simulink model "comparing_controllers"  (R2020a)
settings: Solver=VariableStepAuto  StartTime=0.0  StopTime=50  RelTol=1e-3
libraries: aerolibutil x20, sharedutil x10, slctrlblks x6
(part 1 of 3)
settings Model: Creator=Sebas  LastModifiedBy=Sebas
settings SolverCC: ZeroCrossAlgorithm=Adaptive
settings DebuggingCC: MaskedZcDiagnostic=none  IgnoredZcDiagnostic=none

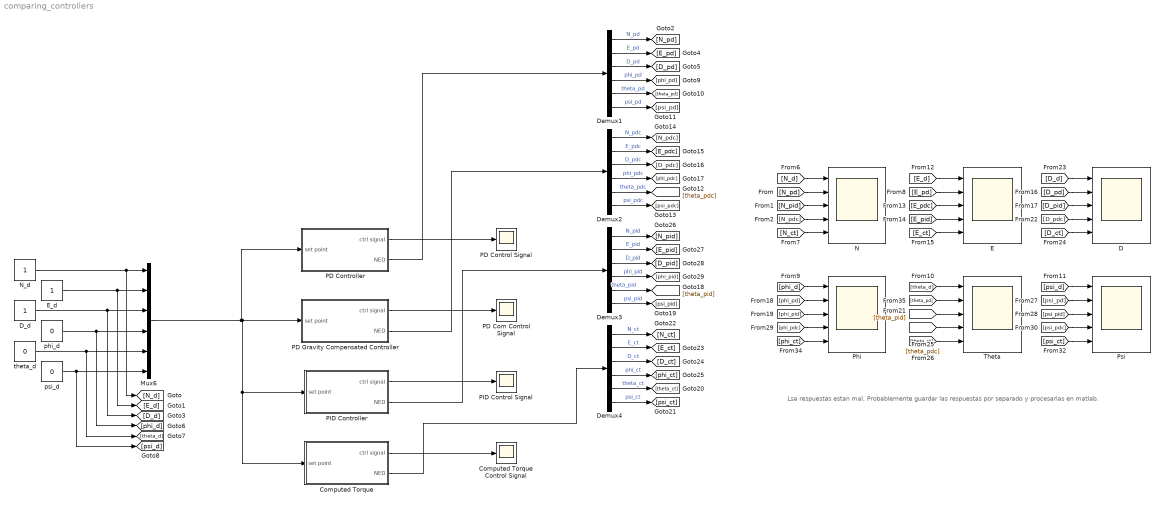
== system comparing_controllers ==
  note: Lsa respuestas estan mal. Probablemente guardar las respuestas por separado y procesarlas en matlab.
  Computed Torque : Subsystem
  Computed Torque Control Signal : Scope
  D : Scope  NumInputPorts=5
  D_d : Constant
  Demux{1..4} (4 alike) : Demux  Outputs=6
  E : Scope  NumInputPorts=5
  E_d : Constant
  Mux6 : Mux  Inputs=6
  N : Scope  NumInputPorts=5
  N_d : Constant
  PD Com Control Signal : Scope
  PD Control Signal : Scope
  PD Controller : Subsystem
  PD Gravity Compensated Controller : Subsystem
  PID Control Signal : Scope
  PID Controller : Subsystem
  Phi : Scope  NumInputPorts=5
  Psi : Scope  NumInputPorts=5
  Theta : Scope  NumInputPorts=5
  phi_d : Constant  Value=0
  psi_d : Constant  Value=0
  theta_d : Constant  Value=0
  wires:
  Demux1/3 -> [D_pd]  "D_pd"
  N_d/1 -> [N_d], Mux6/1
  Demux1/5 -> [theta_pd]  "theta_pd"
  Demux1/1 -> [N_pd]  "N_pd"
  [N_d] -> N/1
  [N_pd] -> N/2
  [N_pid] -> N/3
  D_d/1 -> Mux6/3, [D_d]
  E_d/1 -> [E_d], Mux6/2
  [N_pdc] -> N/4
  Demux1/4 -> [phi_pd]  "phi_pd"
  phi_d/1 -> Mux6/4, [phi_d]
  theta_d/1 -> [theta_d], Mux6/5
  psi_d/1 -> [psi_d], Mux6/6
  Demux1/6 -> [psi_pd]  "psi_pd"
  Demux1/2 -> [E_pd]  "E_pd"
  Mux6/1 -> PD Controller/1(set point), Computed Torque/1(set point), PID Controller/1(set point), PD Gravity Compensated Controller/1(set point)
  PD Controller/1(ctrl signal) -> PD Control Signal/1
  PD Controller/2(NED) -> Demux1/1
  PD Gravity Compensated Controller/1(ctrl signal) -> PD Com Control Signal/1
  PID Controller/1(ctrl signal) -> PID Control Signal/1
  Computed Torque/1(ctrl signal) -> Computed Torque Control Signal/1
  Demux2/6 -> [psi_pdc]  "psi_pdc"
  Demux2/4 -> [phi_pdc]  "phi_pdc"
  Demux2/2 -> [E_pdc]  "E_pdc"
  Demux2/1 -> [N_pdc]  "N_pdc"
  Demux2/5 -> [theta_pdc]  "theta_pdc"
  Demux2/3 -> [D_pdc]  "D_pdc"
  PD Gravity Compensated Controller/2(NED) -> Demux2/1
  Demux3/2 -> [E_pid]  "E_pid"
  Demux3/6 -> [psi_pid]  "psi_pid"
  Demux3/4 -> [phi_pid]  "phi_pid"
  Demux3/1 -> [N_pid]  "N_pid"
  Demux3/5 -> [theta_pid]  "theta_pid"
  Demux3/3 -> [D_pid]  "D_pid"
  Demux4/6 -> [psi_ct]  "psi_ct"
  Demux4/4 -> [phi_ct]  "phi_ct"
  Demux4/1 -> [N_ct]  "N_ct"
  Demux4/5 -> [theta_ct]  "theta_ct"
  Demux4/2 -> [E_ct]  "E_ct"
  Demux4/3 -> [D_ct]  "D_ct"
  PID Controller/2(NED) -> Demux3/1
  Computed Torque/2(NED) -> Demux4/1
  [N_ct] -> N/5
  [E_ct] -> E/5
  [E_pid] -> E/4
  [E_pdc] -> E/3
  [E_pd] -> E/2
  [E_d] -> E/1
  [D_ct] -> D/5
  [D_pd] -> D/2
  [D_pid] -> D/3
  [D_d] -> D/1
  [D_pdc] -> D/4
  [theta_pd] -> Theta/2
  [theta_d] -> Theta/1
  [theta_pdc] -> Theta/4
  [theta_pid] -> Theta/3
  [phi_pdc] -> Phi/4
  [phi_ct] -> Phi/5
  [psi_ct] -> Psi/5
  [psi_pd] -> Psi/2
  [theta_ct] -> Theta/5
  [phi_pd] -> Phi/2
  [psi_pdc] -> Psi/4
  [phi_pid] -> Phi/3
  [psi_d] -> Psi/1
  [psi_pid] -> Psi/3
  [phi_d] -> Phi/1

== system comparing_controllers/Computed Torque ==
  set point : Inport
  Computed Torque Controller : Subsystem
  Terminator : Terminator
  UUV 6DOF Model : Subsystem
  ctrl signal : Outport
  NED : Outport  Port=2
  wires:
  Computed Torque Controller/1(tau) -> ctrl signal/1, UUV 6DOF Model/1(tau)  "ctrl signal"
  UUV 6DOF Model/3(NED) -> NED/1, Computed Torque Controller/2(NED)
  UUV 6DOF Model/1(vel_dot) -> Terminator/1
  set point/1 -> Computed Torque Controller/1(set point)
  UUV 6DOF Model/2(vel) -> Computed Torque Controller/3(vel)

== system comparing_controllers/PD Controller ==
  set point : Inport
  6 DOF PD Controller : Subsystem
  Terminator : Terminator
  Terminator1 : Terminator
  UUV 6DOF Model : Subsystem
  ctrl signal : Outport
  NED : Outport  Port=2
  wires:
  6 DOF PD Controller/1(tau) -> ctrl signal/1, UUV 6DOF Model/1(tau)  "ctrl signal"
  UUV 6DOF Model/2(vel) -> Terminator1/1
  UUV 6DOF Model/3(NED) -> NED/1, 6 DOF PD Controller/2(current)
  UUV 6DOF Model/1(vel_dot) -> Terminator/1
  set point/1 -> 6 DOF PD Controller/1(set point)

== system comparing_controllers/PD Gravity Compensated Controller ==
  set point : Inport
  6 DOF PD Gravity Comp Controller : Subsystem
  Terminator : Terminator
  Terminator1 : Terminator
  UUV 6DOF Model : Subsystem
  ctrl signal : Outport
  NED : Outport  Port=2
  wires:
  UUV 6DOF Model/2(vel) -> Terminator1/1
  UUV 6DOF Model/1(vel_dot) -> Terminator/1
  6 DOF PD Gravity Comp Controller/1(tau) -> ctrl signal/1, UUV 6DOF Model/1(tau)  "ctrl signal"
  UUV 6DOF Model/3(NED) -> NED/1, 6 DOF PD Gravity Comp Controller/2(current)
  set point/1 -> 6 DOF PD Gravity Comp Controller/1(set point)

== system comparing_controllers/PID Controller ==
  set point : Inport
  6 DOF PID Controller : Subsystem
  Terminator : Terminator
  Terminator1 : Terminator
  UUV 6DOF Model : Subsystem
  ctrl signal : Outport
  NED : Outport  Port=2
  wires:
  UUV 6DOF Model/1(vel_dot) -> Terminator/1
  6 DOF PID Controller/1(tau) -> ctrl signal/1, UUV 6DOF Model/1(tau)  "ctrl signal"
  set point/1 -> 6 DOF PID Controller/1(set point)
  UUV 6DOF Model/3(NED) -> NED/1, 6 DOF PID Controller/2(current)
  UUV 6DOF Model/2(vel) -> Terminator1/1

== system comparing_controllers/Computed Torque/Computed Torque Controller ==
  set point : Inport
  NED : Inport  Port=2
  vel : Inport  Port=3
  6 PD + fb linearization Controllers : Subsystem  mask(6 Degrees-of-freedom P-D Controller){surge_kd=0.35, surge_kp=0.7, sway_kd=0.7, sway_kp=0.6, heave_kd=0.2, heave_kp=0.7, roll_kd=1.3, roll_kp=10, pitch_kd=0.05, pitch_kp=0.2, yaw_kd=1.2, yaw_kp=3}
      mask prompts: surge_kd "Surge K derivative"; surge_kp "Surge K proportional"; sway_kd "Sway K derivative"; sway_kp "Sway K proportional"; heave_kd "Heave K derivative"; heave_kp "Heave K proportional"; roll_kd "Roll K derivative"; roll_kp "Roll K proportional"; pitch_kd "Pitch K derivative"; pitch_kp "Pitch K proportional"; yaw_kd "Yaw K derivative"; yaw_kp "Yaw K proportional"
      mask help: Implementation of 6 PD controllers for each degree of freedom
      mask DialogControl ParameterGroupVar Prompt: Gains
  Constant : Constant  Value=0
  Derivative : Derivative  Commented=on
  Derivative1 : Derivative  Commented=on
  Signal Specification : SignalSpecification  Dimensions=6
  Thrust allocation : Subsystem
  Transform : Subsystem
  tau : Outport
  wires:
  Transform/1(Out1) -> 6 PD + fb linearization Controllers/1(set point)  "ideal"
  NED/1 -> Transform/2(NED)
  Signal Specification/1 -> tau/1  "ideal"
  Transform/2(Out2) -> 6 PD + fb linearization Controllers/2(current)  "ideal"
  Thrust allocation/1(tau) -> Signal Specification/1
  6 PD + fb linearization Controllers/1(i_tau) -> Thrust allocation/1(ideal_tau)  "ideal_tau"
  vel/1 -> 6 PD + fb linearization Controllers/3(vel)  "ideal"
  set point/1 -> Transform/1(set point)  "ideal"
  Constant/1 -> 6 PD + fb linearization Controllers/4(vel_dot_d)
  Derivative/1 -> Derivative1/1

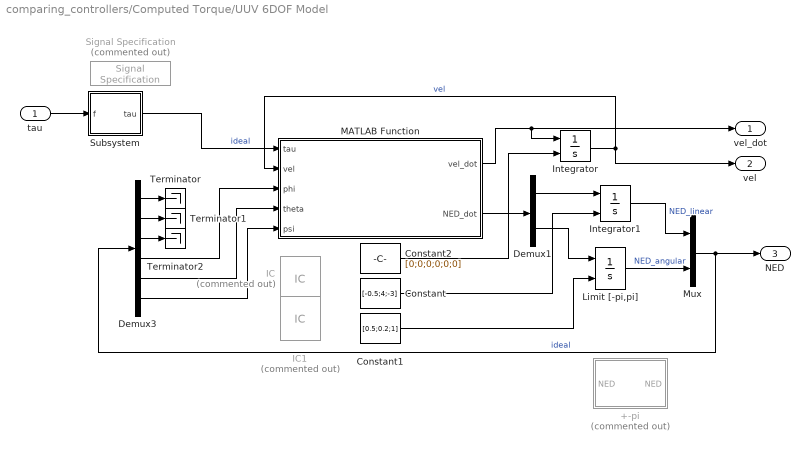
== system comparing_controllers/Computed Torque/UUV 6DOF Model ==
  tau : Inport
  +-pi : MATLAB Function  Commented=on  TreatAsAtomicUnit=on
  Constant : Constant  Value=[-0.5;4;-3]
  Constant1 : Constant  Value=[0.5;0.2;1]
  Constant2 : Constant  Value=[0;0;0;0;0;0]
  Demux1 : Demux  Outputs=2
  Demux3 : Demux  Outputs=6
  IC : InitialCondition  Commented=on  Value=[0;0;0;0;0;0]
  IC1 : InitialCondition  Commented=on  Value=[1;1;1;1;1;1]
  Integrator : Integrator  InitialConditionSource=external
  Integrator1 : Integrator  InitialConditionSource=external
  Limit [-pi,pi] : Integrator  InitialConditionSource=external  WrapState=on
  MATLAB Function : MATLAB Function  TreatAsAtomicUnit=on
  Mux : Mux  Inputs=2
  Signal Specification : SignalSpecification  Commented=on  Dimensions=6
  Subsystem : Subsystem
  Terminator : Terminator
  Terminator1 : Terminator
  Terminator2 : Terminator
  vel_dot : Outport
  vel : Outport  Port=2
  NED : Outport  Port=3
  wires:
  Constant/1 -> Integrator1/2
  Constant1/1 -> Limit [-pi,pi]/2
  Constant2/1 -> Integrator/2
  MATLAB Function/2(NED_dot) -> Demux1/1
  Demux1/1 -> Integrator1/1
  Demux1/2 -> Limit [-pi,pi]/1
  Limit [-pi,pi]/1 -> Mux/2  "NED_angular"
  tau/1 -> Subsystem/1(f)
  Subsystem/1(tau) -> MATLAB Function/1(tau)  "ideal"
  Demux3/3 -> Terminator2/1
  Demux3/1 -> Terminator/1
  Demux3/2 -> Terminator1/1
  Integrator1/1 -> Mux/1  "NED_linear"
  Demux3/6 -> MATLAB Function/5(psi)
  Demux3/5 -> MATLAB Function/4(theta)
  Demux3/4 -> MATLAB Function/3(phi)
  Integrator/1 -> MATLAB Function/2(vel), vel/1  "vel"
  MATLAB Function/1(vel_dot) -> Integrator/1, vel_dot/1
  Mux/1 -> NED/1, Demux3/1  "ideal"

== system comparing_controllers/PD Controller/6 DOF PD Controller ==
  set point : Inport
  current : Inport  Port=2
  6 PD Controllers : Subsystem  mask(6 Degrees-of-freedom P-D Controller){surge_kd=25, surge_kp=15, sway_kd=30, sway_kp=12, heave_kd=7, heave_kp=10, roll_kd=0.6, roll_kp=5, pitch_kd=0, pitch_kp=5, yaw_kd=4.5, yaw_kp=5}
      mask prompts: surge_kd "Surge K derivative"; surge_kp "Surge K proportional"; sway_kd "Sway K derivative"; sway_kp "Sway K proportional"; heave_kd "Heave K derivative"; heave_kp "Heave K proportional"; roll_kd "Roll K derivative"; roll_kp "Roll K proportional"; pitch_kd "Pitch K derivative"; pitch_kp "Pitch K proportional"; yaw_kd "Yaw K derivative"; yaw_kp "Yaw K proportional"
      mask help: Implementation of 6 PD controllers for each degree of freedom
      mask DialogControl ParameterGroupVar Prompt: Gains
  Signal Specification : SignalSpecification  Dimensions=6
  Subsystem : Subsystem  Commented=on
  Thrust allocation : Subsystem
  Transform : Subsystem
  tau : Outport
  wires:
  6 PD Controllers/1(i_tau) -> Thrust allocation/1(ideal_tau)  "ideal_tau"
  Thrust allocation/1(tau) -> Signal Specification/1
  set point/1 -> Transform/1(In1)
  current/1 -> Transform/2(NED)
  Transform/1(Out1) -> 6 PD Controllers/1(set point)
  Transform/2(Out2) -> 6 PD Controllers/2(current)
  Signal Specification/1 -> tau/1  "ideal"

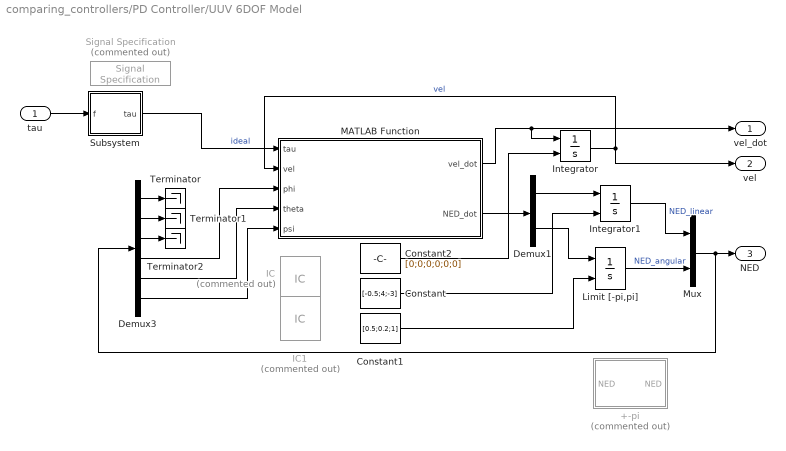
== system comparing_controllers/PD Controller/UUV 6DOF Model ==
  tau : Inport
  +-pi : MATLAB Function  Commented=on  TreatAsAtomicUnit=on
  Constant : Constant  Value=[-0.5;4;-3]
  Constant1 : Constant  Value=[0.5;0.2;1]
  Constant2 : Constant  Value=[0;0;0;0;0;0]
  Demux1 : Demux  Outputs=2
  Demux3 : Demux  Outputs=6
  IC : InitialCondition  Commented=on  Value=[0;0;0;0;0;0]
  IC1 : InitialCondition  Commented=on  Value=[1;1;1;1;1;1]
  Integrator : Integrator  InitialConditionSource=external
  Integrator1 : Integrator  InitialConditionSource=external
  Limit [-pi,pi] : Integrator  InitialConditionSource=external  WrapState=on
  MATLAB Function : MATLAB Function  TreatAsAtomicUnit=on
  Mux : Mux  Inputs=2
  Signal Specification : SignalSpecification  Commented=on  Dimensions=6
  Subsystem : Subsystem
  Terminator : Terminator
  Terminator1 : Terminator
  Terminator2 : Terminator
  vel_dot : Outport
  vel : Outport  Port=2
  NED : Outport  Port=3
  wires:
  Constant/1 -> Integrator1/2
  Constant1/1 -> Limit [-pi,pi]/2
  Constant2/1 -> Integrator/2
  MATLAB Function/2(NED_dot) -> Demux1/1
  Demux1/1 -> Integrator1/1
  Demux1/2 -> Limit [-pi,pi]/1
  Limit [-pi,pi]/1 -> Mux/2  "NED_angular"
  tau/1 -> Subsystem/1(f)
  Subsystem/1(tau) -> MATLAB Function/1(tau)  "ideal"
  Demux3/3 -> Terminator2/1
  Demux3/1 -> Terminator/1
  Demux3/2 -> Terminator1/1
  Integrator1/1 -> Mux/1  "NED_linear"
  Demux3/6 -> MATLAB Function/5(psi)
  Demux3/5 -> MATLAB Function/4(theta)
  Demux3/4 -> MATLAB Function/3(phi)
  Integrator/1 -> MATLAB Function/2(vel), vel/1  "vel"
  Mux/1 -> NED/1, Demux3/1
  MATLAB Function/1(vel_dot) -> Integrator/1, vel_dot/1

== system comparing_controllers/PD Gravity Compensated Controller/6 DOF PD Gravity Comp Controller ==
  set point : Inport
  current : Inport  Port=2
  6 PD Gravity Comp Controllers : Subsystem  mask(6 Degrees-of-freedom P-D and Gravity Compensator Controller){surge_kd=10, surge_kp=5, sway_kd=10, sway_kp=2.5, heave_kd=10, heave_kp=5, roll_kd=30, roll_kp=5, pitch_kd=30, pitch_kp=0.9, yaw_kd=30, yaw_kp=5}
      mask prompts: surge_kd "Surge K derivative"; surge_kp "Surge K proportional"; sway_kd "Sway K derivative"; sway_kp "Sway K proportional"; heave_kd "Heave K derivative"; heave_kp "Heave K proportional"; roll_kd "Roll K derivative"; roll_kp "Roll K proportional"; pitch_kd "Pitch K derivative"; pitch_kp "Pitch K proportional"; yaw_kd "Yaw K derivative"; yaw_kp "Yaw K proportional"
      mask help: Implementation of 6 PD controllers for each degree of freedom plus a Gravity Compensation
      mask DialogControl ParameterGroupVar Prompt: Gains
  Demux6 : Demux  Commented=on  Outputs=3
  Mux2 : Mux  Commented=on  Inputs=3
  Saturation : Saturate  Commented=on  UpperLimit=70  LowerLimit=-70
  Saturation1 : Saturate  Commented=on  UpperLimit=100  LowerLimit=-100
  Saturation2 : Saturate  Commented=on  UpperLimit=100  LowerLimit=-100
  Signal Specification : SignalSpecification  Dimensions=6
  Subsystem : Subsystem  Commented=on
  Subsystem3 : Subsystem  Commented=on
  Thrust allocation : Subsystem
  Transform : Subsystem
  tau : Outport
  wires:
  6 PD Gravity Comp Controllers/1(i_tau) -> Thrust allocation/1(ideal_tau)  "ideal_tau"
  Thrust allocation/1(tau) -> Signal Specification/1  "ideal_t_sat"
  set point/1 -> Transform/1(In1)
  current/1 -> Transform/2(NED)
  Transform/1(Out1) -> 6 PD Gravity Comp Controllers/1(set point)
  Transform/2(Out2) -> 6 PD Gravity Comp Controllers/2(current)
  Saturation1/1 -> Mux2/1
  Saturation/1 -> Mux2/3
  Demux6/2 -> Saturation2/1
  Demux6/1 -> Saturation1/1
  Saturation2/1 -> Mux2/2
  Demux6/3 -> Saturation/1
  Signal Specification/1 -> tau/1  "ideal"

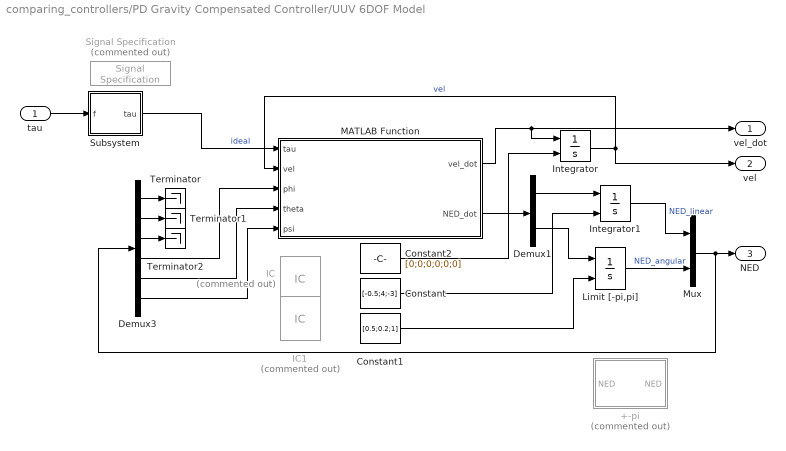
== system comparing_controllers/PD Gravity Compensated Controller/UUV 6DOF Model ==
  tau : Inport
  +-pi : MATLAB Function  Commented=on  TreatAsAtomicUnit=on
  Constant : Constant  Value=[-0.5;4;-3]
  Constant1 : Constant  Value=[0.5;0.2;1]
  Constant2 : Constant  Value=[0;0;0;0;0;0]
  Demux1 : Demux  Outputs=2
  Demux3 : Demux  Outputs=6
  IC : InitialCondition  Commented=on  Value=[0;0;0;0;0;0]
  IC1 : InitialCondition  Commented=on  Value=[1;1;1;1;1;1]
  Integrator : Integrator  InitialConditionSource=external
  Integrator1 : Integrator  InitialConditionSource=external
  Limit [-pi,pi] : Integrator  InitialConditionSource=external  WrapState=on
  MATLAB Function : MATLAB Function  TreatAsAtomicUnit=on
  Mux : Mux  Inputs=2
  Signal Specification : SignalSpecification  Commented=on  Dimensions=6
  Subsystem : Subsystem
  Terminator : Terminator
  Terminator1 : Terminator
  Terminator2 : Terminator
  vel_dot : Outport
  vel : Outport  Port=2
  NED : Outport  Port=3
  wires:
  Constant/1 -> Integrator1/2
  Constant1/1 -> Limit [-pi,pi]/2
  Constant2/1 -> Integrator/2
  MATLAB Function/2(NED_dot) -> Demux1/1
  Demux1/1 -> Integrator1/1
  Demux1/2 -> Limit [-pi,pi]/1
  Limit [-pi,pi]/1 -> Mux/2  "NED_angular"
  tau/1 -> Subsystem/1(f)
  Subsystem/1(tau) -> MATLAB Function/1(tau)  "ideal"
  Demux3/3 -> Terminator2/1
  Demux3/1 -> Terminator/1
  Demux3/2 -> Terminator1/1
  Integrator1/1 -> Mux/1  "NED_linear"
  Demux3/6 -> MATLAB Function/5(psi)
  Demux3/5 -> MATLAB Function/4(theta)
  Demux3/4 -> MATLAB Function/3(phi)
  Integrator/1 -> MATLAB Function/2(vel), vel/1  "vel"
  Mux/1 -> NED/1, Demux3/1
  MATLAB Function/1(vel_dot) -> Integrator/1, vel_dot/1

== system comparing_controllers/PID Controller/6 DOF PID Controller ==
  set point : Inport
  current : Inport  Port=2
  6 PID Controllers : Subsystem  mask(6 Degrees-of-freedom P-I-D Controller){surge_kd=22, surge_kp=13, surge_ki=0, sway_kd=22, sway_kp=7, sway_ki=0, heave_kd=15, heave_kp=7, heave_ki=0.18, roll_kd=0.6, roll_kp=5, roll_ki=0.1, pitch_kd=0, pitch_kp=5, pitch_ki=0.1, yaw_kd=4.5, yaw_kp=5, yaw_ki=0}
      mask prompts: surge_kd "Surge K derivative"; surge_kp "Surge K proportional"; surge_ki "Surge K integral"; sway_kd "Sway K derivative"; sway_kp "Sway K proportional"; sway_ki "Sway K integral"; heave_kd "Heave K derivative"; heave_kp "Heave K proportional"; heave_ki "Heave K integral"; roll_kd "Roll K derivative"; roll_kp "Roll K proportional"; roll_ki "Roll K integral"; pitch_kd "Pitch K derivative"; pitch_kp "Pitch K proportional"; pitch_ki "Pitch K integral"; yaw_kd "Yaw K derivative"; yaw_kp "Yaw K proportional"; yaw_ki "Yaw K integral"
      mask help: Implementation of 6 PID controllers for each degree of freedom
      mask DialogControl ParameterGroupVar Prompt: Gains
  Signal Specification : SignalSpecification  Dimensions=6
  Thrust allocation : Subsystem
  Transform : Subsystem
  tau : Outport
  wires:
  Transform/2(Out2) -> 6 PID Controllers/2(current)
  Thrust allocation/1(tau) -> Signal Specification/1
  Transform/1(Out1) -> 6 PID Controllers/1(set point)
  6 PID Controllers/1(i_tau) -> Thrust allocation/1(ideal_tau)  "ideal_tau"
  Signal Specification/1 -> tau/1  "ideal"
  set point/1 -> Transform/1(set point)
  current/1 -> Transform/2(NED)

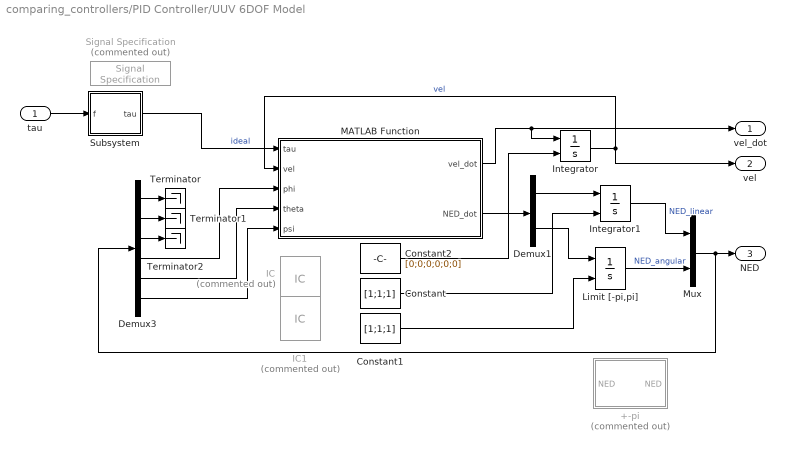
== system comparing_controllers/PID Controller/UUV 6DOF Model ==
  tau : Inport
  +-pi : MATLAB Function  Commented=on  TreatAsAtomicUnit=on
  Constant : Constant  Value=[1;1;1]
  Constant1 : Constant  Value=[1;1;1]
  Constant2 : Constant  Value=[0;0;0;0;0;0]
  Demux1 : Demux  Outputs=2
  Demux3 : Demux  Outputs=6
  IC : InitialCondition  Commented=on  Value=[0;0;0;0;0;0]
  IC1 : InitialCondition  Commented=on  Value=[1;1;1;1;1;1]
  Integrator : Integrator  InitialConditionSource=external
  Integrator1 : Integrator  InitialConditionSource=external
  Limit [-pi,pi] : Integrator  InitialConditionSource=external  WrapState=on
  MATLAB Function : MATLAB Function  TreatAsAtomicUnit=on
  Mux : Mux  Inputs=2
  Signal Specification : SignalSpecification  Commented=on  Dimensions=6
  Subsystem : Subsystem
  Terminator : Terminator
  Terminator1 : Terminator
  Terminator2 : Terminator
  vel_dot : Outport
  vel : Outport  Port=2
  NED : Outport  Port=3
  wires:
  Constant/1 -> Integrator1/2
  Constant1/1 -> Limit [-pi,pi]/2
  Constant2/1 -> Integrator/2
  MATLAB Function/2(NED_dot) -> Demux1/1
  Demux1/1 -> Integrator1/1
  Demux1/2 -> Limit [-pi,pi]/1
  Limit [-pi,pi]/1 -> Mux/2  "NED_angular"
  tau/1 -> Subsystem/1(f)
  Subsystem/1(tau) -> MATLAB Function/1(tau)  "ideal"
  Demux3/3 -> Terminator2/1
  Demux3/1 -> Terminator/1
  Demux3/2 -> Terminator1/1
  Integrator1/1 -> Mux/1  "NED_linear"
  Demux3/6 -> MATLAB Function/5(psi)
  Demux3/5 -> MATLAB Function/4(theta)
  Demux3/4 -> MATLAB Function/3(phi)
  Integrator/1 -> MATLAB Function/2(vel), vel/1  "vel"
  Mux/1 -> NED/1, Demux3/1
  MATLAB Function/1(vel_dot) -> Integrator/1, vel_dot/1

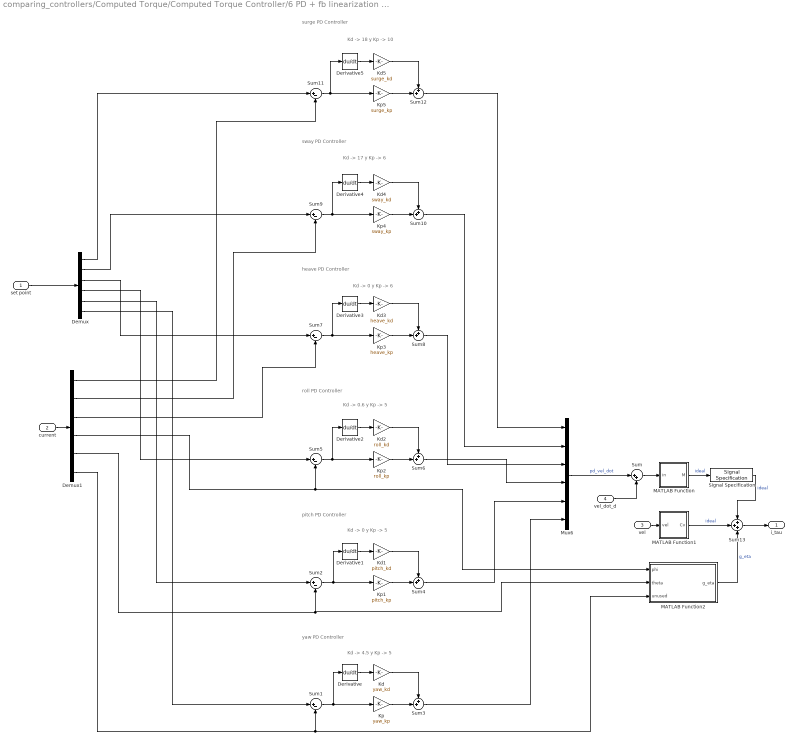
== system comparing_controllers/Computed Torque/Computed Torque Controller/6 PD + fb linearization Controllers ==
  note: surge PD Controller
  note: sway PD Controller
  note: heave PD Controller
  note: roll PD Controller
  note: pitch PD Controller
  note: yaw PD Controller
  note: Kd -> 4.5 y Kp -> 5
  note: Kd -> 0 y Kp -> 5
  note: Kd -> 0.6 y Kp -> 5
  note: Kd -> 0 y Kp -> 6
  note: Kd -> 17 y Kp -> 6
  note: Kd -> 18 y Kp -> 10
  set point : Inport
  current : Inport  Port=2
  vel : Inport  Port=3
  vel_dot_d : Inport  Port=4
  Demux : Demux  Outputs=6
  Demux1 : Demux  Outputs=6
  Derivative{,1..5} (6 alike) : Derivative
  Kd : Gain  Gain=yaw_kd
  Kd1 : Gain  Gain=pitch_kd
  Kd2 : Gain  Gain=roll_kd
  Kd3 : Gain  Gain=heave_kd
  Kd4 : Gain  Gain=sway_kd
  Kd5 : Gain  Gain=surge_kd
  Kp : Gain  Gain=yaw_kp
  Kp1 : Gain  Gain=pitch_kp
  Kp2 : Gain  Gain=roll_kp
  Kp3 : Gain  Gain=heave_kp
  Kp4 : Gain  Gain=sway_kp
  Kp5 : Gain  Gain=surge_kp
  MATLAB Function : MATLAB Function  TreatAsAtomicUnit=on
  MATLAB Function1 : MATLAB Function  TreatAsAtomicUnit=on
  MATLAB Function2 : MATLAB Function  TreatAsAtomicUnit=on
  Mux6 : Mux  Inputs=6
  Signal Specification : SignalSpecification  Dimensions=6
  Sum : Sum  Inputs=|++
  Sum{1..2,5,7,9,11} (6 alike) : Sum  Inputs=|+-
  Sum{3..4,6,8,10,12} (6 alike) : Sum  Inputs=++|
  Sum13 : Sum  Inputs=+++
  i_tau : Outport
  wires:
  Sum8/1 -> Mux6/3
  Sum4/1 -> Mux6/5
  Sum6/1 -> Mux6/4
  Sum3/1 -> Mux6/6
  Sum12/1 -> Mux6/1
  Sum10/1 -> Mux6/2
  Derivative/1 -> Kd/1
  Kp/1 -> Sum3/2
  Kd/1 -> Sum3/1
  Sum1/1 -> Derivative/1, Kp/1
  Sum2/1 -> Kp1/1, Derivative1/1
  Kd1/1 -> Sum4/1
  Kp1/1 -> Sum4/2
  Derivative1/1 -> Kd1/1
  Derivative2/1 -> Kd2/1
  Kp2/1 -> Sum6/2
  Kd2/1 -> Sum6/1
  Sum5/1 -> Derivative2/1, Kp2/1
  Derivative3/1 -> Kd3/1
  Kp3/1 -> Sum8/2
  Kd3/1 -> Sum8/1
  Sum7/1 -> Derivative3/1, Kp3/1
  Derivative4/1 -> Kd4/1
  Kp4/1 -> Sum10/2
  Kd4/1 -> Sum10/1
  Sum9/1 -> Derivative4/1, Kp4/1
  Derivative5/1 -> Kd5/1
  Kp5/1 -> Sum12/2
  Kd5/1 -> Sum12/1
  Sum11/1 -> Derivative5/1, Kp5/1
  current/1 -> Demux1/1
  Demux1/1 -> Sum11/2
  set point/1 -> Demux/1
  Demux/1 -> Sum11/1
  Demux/2 -> Sum9/1
  Demux1/2 -> Sum9/2
  Demux/3 -> Sum7/1
  Demux1/3 -> Sum7/2
  Demux/4 -> Sum5/1
  Demux1/4 -> MATLAB Function2/1(phi), Sum5/2
  Demux/5 -> Sum2/1
  Demux1/5 -> MATLAB Function2/2(theta), Sum2/2
  Demux/6 -> Sum1/1
  Demux1/6 -> MATLAB Function2/3(unused), Sum1/2
  Mux6/1 -> Sum/1  "pd_vel_dot"
  Sum/1 -> MATLAB Function/1(in)
  vel_dot_d/1 -> Sum/2
  Sum13/1 -> i_tau/1
  vel/1 -> MATLAB Function1/1(vel)
  MATLAB Function/1(M) -> Signal Specification/1  "ideal"
  MATLAB Function2/1(g_eta) -> Sum13/3  "g_eta"
  MATLAB Function1/1(Cv) -> Sum13/2  "ideal"
  Signal Specification/1 -> Sum13/1  "ideal"

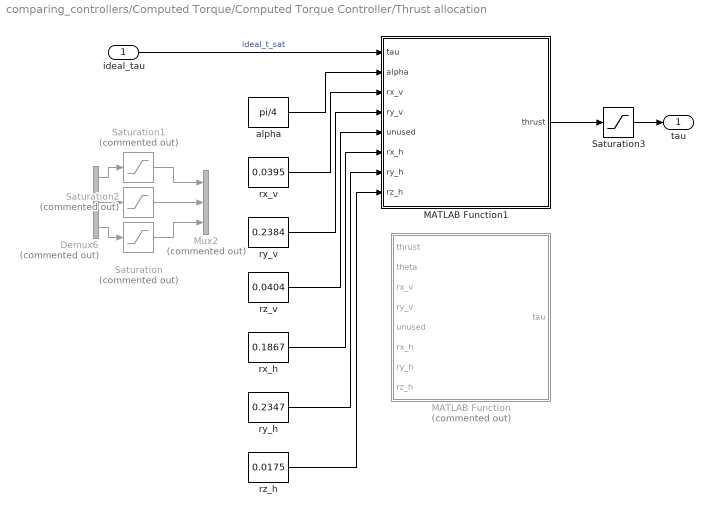
== system comparing_controllers/Computed Torque/Computed Torque Controller/Thrust allocation ==
  ideal_tau : Inport
  Demux6 : Demux  Commented=on  Outputs=3
  MATLAB Function : MATLAB Function  Commented=on  TreatAsAtomicUnit=on
  MATLAB Function1 : MATLAB Function  TreatAsAtomicUnit=on
  Mux2 : Mux  Commented=on  Inputs=3
  Saturation : Saturate  Commented=on  UpperLimit=70  LowerLimit=-70
  Saturation1 : Saturate  Commented=on  UpperLimit=100  LowerLimit=-100
  Saturation2 : Saturate  Commented=on  UpperLimit=100  LowerLimit=-100
  Saturation3 : Saturate  UpperLimit=35  LowerLimit=-35
  alpha : Constant  Value=pi/4
  rx_h : Constant  Value=0.1867
  rx_v : Constant  Value=0.0395
  ry_h : Constant  Value=0.2347
  ry_v : Constant  Value=0.2384
  rz_h : Constant  Value=0.0175
  rz_v : Constant  Value=0.0404
  tau : Outport
  wires:
  ideal_tau/1 -> MATLAB Function1/1(tau)  "ideal_t_sat"
  MATLAB Function1/1(thrust) -> Saturation3/1
  Saturation3/1 -> tau/1
  rx_v/1 -> MATLAB Function1/3(rx_v)
  alpha/1 -> MATLAB Function1/2(alpha)
  rx_h/1 -> MATLAB Function1/6(rx_h)
  ry_h/1 -> MATLAB Function1/7(ry_h)
  rz_h/1 -> MATLAB Function1/8(rz_h)
  ry_v/1 -> MATLAB Function1/4(ry_v)
  rz_v/1 -> MATLAB Function1/5(unused)
  Demux6/2 -> Saturation2/1
  Demux6/3 -> Saturation/1
  Saturation1/1 -> Mux2/1
  Saturation/1 -> Mux2/3
  Demux6/1 -> Saturation1/1
  Saturation2/1 -> Mux2/2

== system comparing_controllers/Computed Torque/Computed Torque Controller/Transform ==
  set point : Inport
  NED : Inport  Port=2
  Demux : Demux  Outputs=2
  Demux1 : Demux  Outputs=2
  Mux1 : Mux  Inputs=2
  Mux2 : Mux  Inputs=2
  Mux3 : Mux  Inputs=2
  Subsystem1 : Subsystem
  Subsystem2 : Subsystem
  Terminator5 : Terminator
  Out1 : Outport
  Out2 : Outport  Port=2
  wires:
  Demux/1 -> Mux2/1
  NED/1 -> Demux1/1, Subsystem1/1(NED)
  set point/1 -> Demux/1
  Demux/2 -> Mux1/2
  Subsystem2/1(pos_body) -> Mux1/1
  Demux1/1 -> Terminator5/1
  Subsystem1/1(pos_body) -> Mux3/1
  Demux1/2 -> Mux2/2, Mux3/2
  Mux2/1 -> Subsystem2/1(NED)
  Mux3/1 -> Out2/1
  Mux1/1 -> Out1/1

== system comparing_controllers/Computed Torque/UUV 6DOF Model/Subsystem ==
  f : Inport
  MATLAB Function1 : MATLAB Function  TreatAsAtomicUnit=on
  rx_h : Constant  Value=0.1867
  rx_v : Constant  Value=0.0395
  ry_h : Constant  Value=0.2347
  ry_v : Constant  Value=0.2384
  rz_h : Constant  Value=0.0175
  rz_v : Constant  Value=0.0404
  theta : Constant  Value=pi/4
  tau : Outport
  wires:
  rz_v/1 -> MATLAB Function1/5(unused)
  ry_h/1 -> MATLAB Function1/7(ry_h)
  f/1 -> MATLAB Function1/1(f)
  MATLAB Function1/1(tau) -> tau/1
  rx_h/1 -> MATLAB Function1/6(rx_h)
  theta/1 -> MATLAB Function1/2(theta)
  rx_v/1 -> MATLAB Function1/3(rx_v)
  rz_h/1 -> MATLAB Function1/8(rz_h)
  ry_v/1 -> MATLAB Function1/4(ry_v)

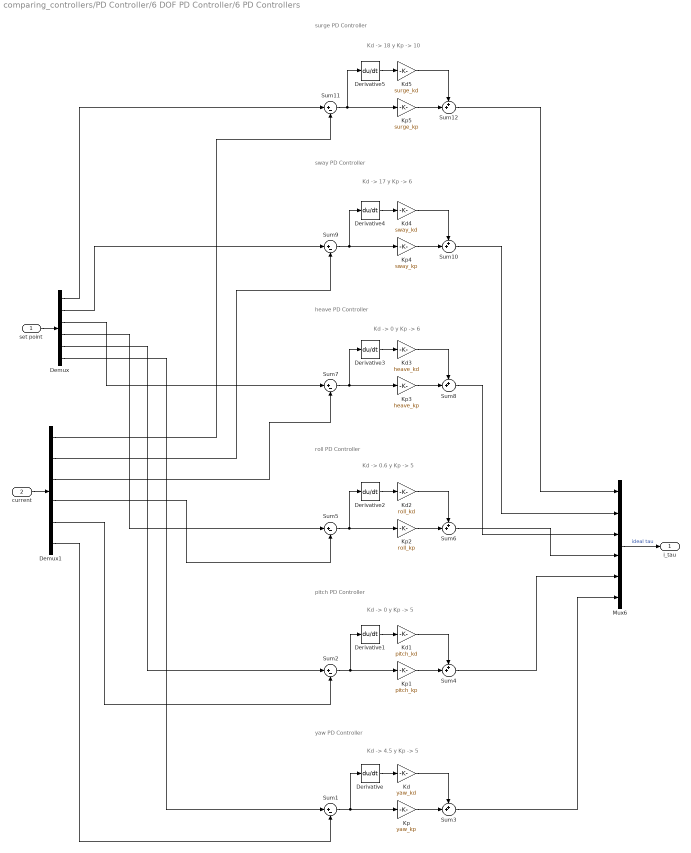
== system comparing_controllers/PD Controller/6 DOF PD Controller/6 PD Controllers ==
  note: surge PD Controller
  note: sway PD Controller
  note: heave PD Controller
  note: roll PD Controller
  note: pitch PD Controller
  note: yaw PD Controller
  note: Kd -> 4.5 y Kp -> 5
  note: Kd -> 0 y Kp -> 5
  note: Kd -> 0.6 y Kp -> 5
  note: Kd -> 0 y Kp -> 6
  note: Kd -> 17 y Kp -> 6
  note: Kd -> 18 y Kp -> 10
  set point : Inport
  current : Inport  Port=2
  Demux : Demux  Outputs=6
  Demux1 : Demux  Outputs=6
  Derivative{,1..5} (6 alike) : Derivative
  Kd : Gain  Gain=yaw_kd
  Kd1 : Gain  Gain=pitch_kd
  Kd2 : Gain  Gain=roll_kd
  Kd3 : Gain  Gain=heave_kd
  Kd4 : Gain  Gain=sway_kd
  Kd5 : Gain  Gain=surge_kd
  Kp : Gain  Gain=yaw_kp
  Kp1 : Gain  Gain=pitch_kp
  Kp2 : Gain  Gain=roll_kp
  Kp3 : Gain  Gain=heave_kp
  Kp4 : Gain  Gain=sway_kp
  Kp5 : Gain  Gain=surge_kp
  Mux6 : Mux  Inputs=6
  Sum{1..2,5,7,9,11} (6 alike) : Sum  Inputs=|+-
  Sum{3..4,6,8,10,12} (6 alike) : Sum  Inputs=++|
  i_tau : Outport
  wires:
  Sum8/1 -> Mux6/3
  Sum4/1 -> Mux6/5
  Sum6/1 -> Mux6/4
  Sum3/1 -> Mux6/6
  Sum12/1 -> Mux6/1
  Sum10/1 -> Mux6/2
  Derivative/1 -> Kd/1
  Kp/1 -> Sum3/2
  Kd/1 -> Sum3/1
  Sum1/1 -> Derivative/1, Kp/1
  Sum2/1 -> Kp1/1, Derivative1/1
  Kd1/1 -> Sum4/1
  Kp1/1 -> Sum4/2
  Derivative1/1 -> Kd1/1
  Derivative2/1 -> Kd2/1
  Kp2/1 -> Sum6/2
  Kd2/1 -> Sum6/1
  Sum5/1 -> Derivative2/1, Kp2/1
  Derivative3/1 -> Kd3/1
  Kp3/1 -> Sum8/2
  Kd3/1 -> Sum8/1
  Sum7/1 -> Derivative3/1, Kp3/1
  Derivative4/1 -> Kd4/1
  Kp4/1 -> Sum10/2
  Kd4/1 -> Sum10/1
  Sum9/1 -> Derivative4/1, Kp4/1
  Derivative5/1 -> Kd5/1
  Kp5/1 -> Sum12/2
  Kd5/1 -> Sum12/1
  Sum11/1 -> Derivative5/1, Kp5/1
  current/1 -> Demux1/1
  Demux1/1 -> Sum11/2
  set point/1 -> Demux/1
  Demux/1 -> Sum11/1
  Demux/2 -> Sum9/1
  Demux1/2 -> Sum9/2
  Demux/3 -> Sum7/1
  Demux1/3 -> Sum7/2
  Demux/4 -> Sum5/1
  Demux1/4 -> Sum5/2
  Demux/5 -> Sum2/1
  Demux1/5 -> Sum2/2
  Demux/6 -> Sum1/1
  Demux1/6 -> Sum1/2
  Mux6/1 -> i_tau/1  "ideal tau"

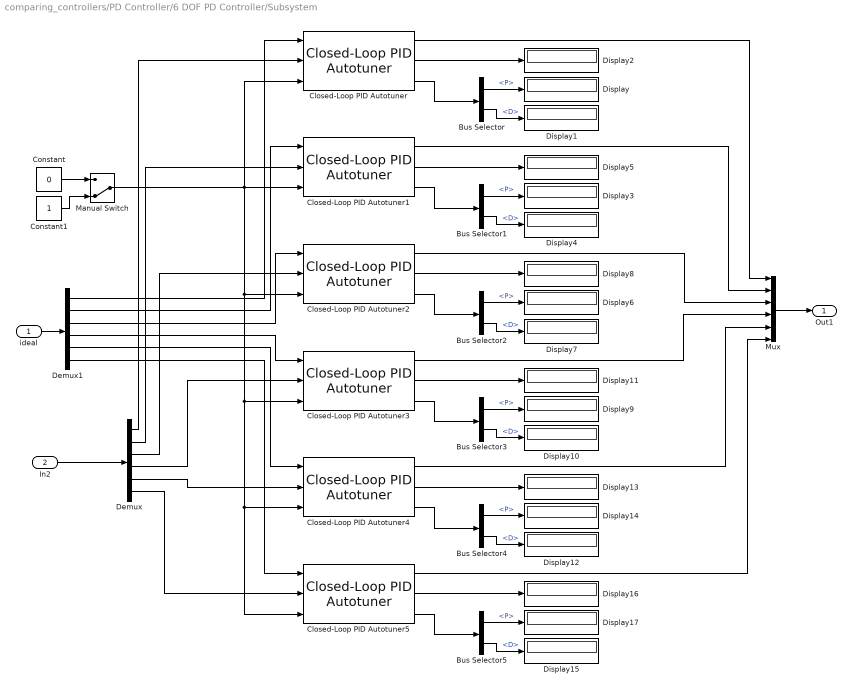
== system comparing_controllers/PD Controller/6 DOF PD Controller/Subsystem ==
  ideal : Inport
  In2 : Inport  Port=2
  Bus Selector{,1..5} (6 alike) : BusSelector  OutputSignals=P,D
  Closed-Loop PID Autotuner{,1..5} (6 alike) : slctrlblks/Closed-Loop PID Autotuner  PIDType=PD  PIDForm=Parallel  TimeDomain=continuous-time  DiscreteTs=0.1  IntegratorFormula=Forward Euler  FilterFormula=Forward Euler  ContinuousTs=0.02  Bandwidth=2/10  UseExternalWC=off  TargetPM=60  UseExternalPM=off  UseExternalAchievedPM=off  PlantType=Integrating  PlantSign=Positive  AmpSine=35  UseExternalAmpSine=off  UseExternalFRD=off  UseExternalU0=off  UseCompanion=off  NotDeployTuningModule=off  UsePLCCoder=off  OutputMode=control action + perturbation  BlockDataType=double  UseConnectedPID=on  blockpath=[]  tunedP=0  tunedI=0  tunedD=0  tunedN=100  tunedPM=0  EstimationWindowSize=3  UseExternalTuningParams=off  OutputChoice=VariantCandD
      settings: SourceProductBaseCode=SD
  Constant : Constant  Value=0
  Constant1 : Constant
  Demux : Demux  Outputs=6
  Demux1 : Demux  Outputs=6
  Display{,1..17} (18 alike) : Display
  Manual Switch : ManualSwitch  CurrentSetting=0
  Mux : Mux  Inputs=6
  Out1 : Outport
  wires:
  Closed-Loop PID Autotuner2/3 -> Bus Selector2/1
  Closed-Loop PID Autotuner/2 -> Display2/1
  Constant/1 -> Manual Switch/1
  Demux/4 -> Closed-Loop PID Autotuner3/2
  Closed-Loop PID Autotuner/3 -> Bus Selector/1
  Manual Switch/1 -> Closed-Loop PID Autotuner/3, Closed-Loop PID Autotuner5/3, Closed-Loop PID Autotuner4/3, Closed-Loop PID Autotuner3/3, Closed-Loop PID Autotuner2/3, Closed-Loop PID Autotuner1/3
  Closed-Loop PID Autotuner2/1 -> Mux/3
  Closed-Loop PID Autotuner4/2 -> Display13/1
  Bus Selector3/1 -> Display9/1  "<P>"
  Bus Selector4/1 -> Display14/1  "<P>"
  Closed-Loop PID Autotuner3/3 -> Bus Selector3/1
  Bus Selector1/2 -> Display4/1  "<D>"
  Constant1/1 -> Manual Switch/2
  Demux1/1 -> Closed-Loop PID Autotuner/1
  Bus Selector/1 -> Display/1  "<P>"
  Closed-Loop PID Autotuner3/2 -> Display11/1
  ideal/1 -> Demux1/1
  Demux1/6 -> Closed-Loop PID Autotuner5/1
  Demux1/5 -> Closed-Loop PID Autotuner4/1
  Bus Selector3/2 -> Display10/1  "<D>"
  Closed-Loop PID Autotuner1/2 -> Display5/1
  Demux1/4 -> Closed-Loop PID Autotuner3/1
  Bus Selector/2 -> Display1/1  "<D>"
  Demux/2 -> Closed-Loop PID Autotuner1/2
  Demux1/3 -> Closed-Loop PID Autotuner2/1
  Closed-Loop PID Autotuner1/1 -> Mux/2
  Closed-Loop PID Autotuner5/2 -> Display16/1
  Bus Selector4/2 -> Display12/1  "<D>"
  Bus Selector1/1 -> Display3/1  "<P>"
  Closed-Loop PID Autotuner1/3 -> Bus Selector1/1
  Demux1/2 -> Closed-Loop PID Autotuner1/1
  Closed-Loop PID Autotuner5/1 -> Mux/6
  Closed-Loop PID Autotuner4/1 -> Mux/5
  Closed-Loop PID Autotuner3/1 -> Mux/4
  In2/1 -> Demux/1
  Closed-Loop PID Autotuner5/3 -> Bus Selector5/1
  Closed-Loop PID Autotuner/1 -> Mux/1
  Bus Selector5/1 -> Display17/1  "<P>"
  Demux/3 -> Closed-Loop PID Autotuner2/2
  Bus Selector5/2 -> Display15/1  "<D>"
  Demux/5 -> Closed-Loop PID Autotuner4/2
  Bus Selector2/2 -> Display7/1  "<D>"
  Demux/1 -> Closed-Loop PID Autotuner/2
  Bus Selector2/1 -> Display6/1  "<P>"
  Closed-Loop PID Autotuner2/2 -> Display8/1
  Closed-Loop PID Autotuner4/3 -> Bus Selector4/1
  Demux/6 -> Closed-Loop PID Autotuner5/2
  Mux/1 -> Out1/1

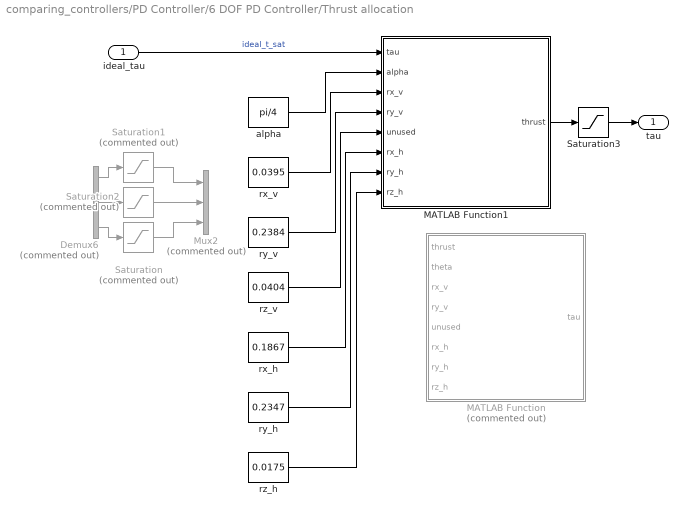
== system comparing_controllers/PD Controller/6 DOF PD Controller/Thrust allocation ==
  ideal_tau : Inport
  Demux6 : Demux  Commented=on  Outputs=3
  MATLAB Function : MATLAB Function  Commented=on  TreatAsAtomicUnit=on
  MATLAB Function1 : MATLAB Function  TreatAsAtomicUnit=on
  Mux2 : Mux  Commented=on  Inputs=3
  Saturation : Saturate  Commented=on  UpperLimit=70  LowerLimit=-70
  Saturation1 : Saturate  Commented=on  UpperLimit=100  LowerLimit=-100
  Saturation2 : Saturate  Commented=on  UpperLimit=100  LowerLimit=-100
  Saturation3 : Saturate  UpperLimit=35  LowerLimit=-35
  alpha : Constant  Value=pi/4
  rx_h : Constant  Value=0.1867
  rx_v : Constant  Value=0.0395
  ry_h : Constant  Value=0.2347
  ry_v : Constant  Value=0.2384
  rz_h : Constant  Value=0.0175
  rz_v : Constant  Value=0.0404
  tau : Outport
  wires:
  ideal_tau/1 -> MATLAB Function1/1(tau)  "ideal_t_sat"
  MATLAB Function1/1(thrust) -> Saturation3/1
  Saturation3/1 -> tau/1
  rx_v/1 -> MATLAB Function1/3(rx_v)
  alpha/1 -> MATLAB Function1/2(alpha)
  rx_h/1 -> MATLAB Function1/6(rx_h)
  ry_h/1 -> MATLAB Function1/7(ry_h)
  rz_h/1 -> MATLAB Function1/8(rz_h)
  ry_v/1 -> MATLAB Function1/4(ry_v)
  rz_v/1 -> MATLAB Function1/5(unused)
  Demux6/2 -> Saturation2/1
  Demux6/3 -> Saturation/1
  Saturation1/1 -> Mux2/1
  Saturation/1 -> Mux2/3
  Demux6/1 -> Saturation1/1
  Saturation2/1 -> Mux2/2

== system comparing_controllers/PD Controller/6 DOF PD Controller/Transform ==
  In1 : Inport
  NED : Inport  Port=2
  Demux : Demux  Outputs=2
  Demux1 : Demux  Outputs=2
  Mux1 : Mux  Inputs=2
  Mux2 : Mux  Inputs=2
  Mux3 : Mux  Inputs=2
  Subsystem1 : Subsystem
  Subsystem2 : Subsystem
  Terminator5 : Terminator
  Out1 : Outport
  Out2 : Outport  Port=2
  wires:
  Demux/1 -> Mux2/1
  NED/1 -> Demux1/1, Subsystem1/1(NED)
  In1/1 -> Demux/1
  Demux/2 -> Mux1/2
  Subsystem2/1(pos_body) -> Mux1/1
  Demux1/1 -> Terminator5/1
  Subsystem1/1(pos_body) -> Mux3/1
  Demux1/2 -> Mux2/2, Mux3/2
  Mux2/1 -> Subsystem2/1(NED)
  Mux3/1 -> Out2/1
  Mux1/1 -> Out1/1

== system comparing_controllers/PD Controller/UUV 6DOF Model/Subsystem ==
  f : Inport
  MATLAB Function1 : MATLAB Function  TreatAsAtomicUnit=on
  rx_h : Constant  Value=0.1867
  rx_v : Constant  Value=0.0395
  ry_h : Constant  Value=0.2347
  ry_v : Constant  Value=0.2384
  rz_h : Constant  Value=0.0175
  rz_v : Constant  Value=0.0404
  theta : Constant  Value=pi/4
  tau : Outport
  wires:
  rz_v/1 -> MATLAB Function1/5(unused)
  ry_h/1 -> MATLAB Function1/7(ry_h)
  f/1 -> MATLAB Function1/1(f)
  MATLAB Function1/1(tau) -> tau/1
  rx_h/1 -> MATLAB Function1/6(rx_h)
  theta/1 -> MATLAB Function1/2(theta)
  rx_v/1 -> MATLAB Function1/3(rx_v)
  rz_h/1 -> MATLAB Function1/8(rz_h)
  ry_v/1 -> MATLAB Function1/4(ry_v)

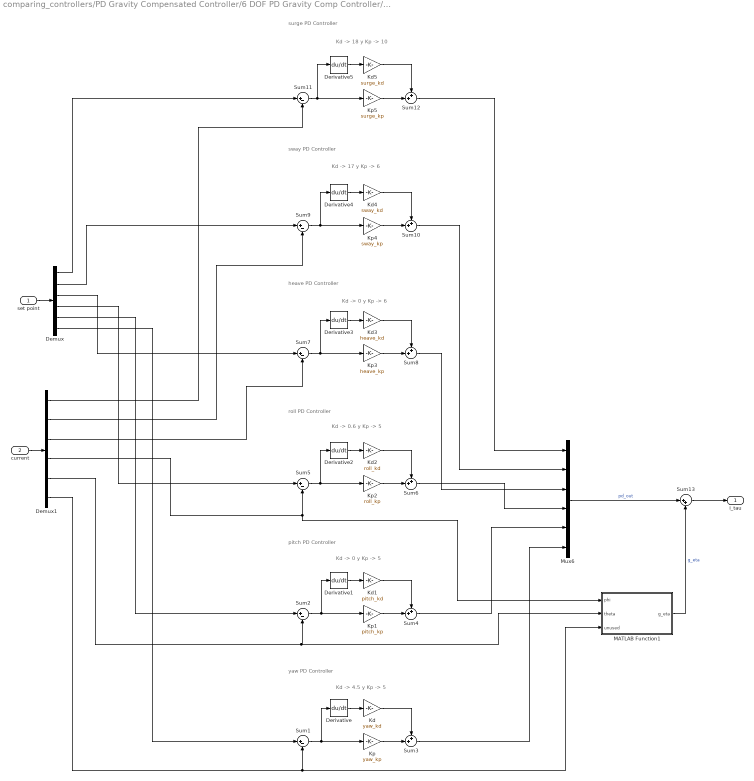
== system comparing_controllers/PD Gravity Compensated Controller/6 DOF PD Gravity Comp Controller/6 PD Gravity Comp Controllers ==
  note: surge PD Controller
  note: sway PD Controller
  note: heave PD Controller
  note: roll PD Controller
  note: pitch PD Controller
  note: yaw PD Controller
  note: Kd -> 4.5 y Kp -> 5
  note: Kd -> 0 y Kp -> 5
  note: Kd -> 0.6 y Kp -> 5
  note: Kd -> 0 y Kp -> 6
  note: Kd -> 17 y Kp -> 6
  note: Kd -> 18 y Kp -> 10
  set point : Inport
  current : Inport  Port=2
  Demux : Demux  Outputs=6
  Demux1 : Demux  Outputs=6
  Derivative{,1..5} (6 alike) : Derivative
  Kd : Gain  Gain=yaw_kd
  Kd1 : Gain  Gain=pitch_kd
  Kd2 : Gain  Gain=roll_kd
  Kd3 : Gain  Gain=heave_kd
  Kd4 : Gain  Gain=sway_kd
  Kd5 : Gain  Gain=surge_kd
  Kp : Gain  Gain=yaw_kp
  Kp1 : Gain  Gain=pitch_kp
  Kp2 : Gain  Gain=roll_kp
  Kp3 : Gain  Gain=heave_kp
  Kp4 : Gain  Gain=sway_kp
  Kp5 : Gain  Gain=surge_kp
  MATLAB Function1 : MATLAB Function  TreatAsAtomicUnit=on
  Mux6 : Mux  Inputs=6
  Sum{1..2,5,7,9,11} (6 alike) : Sum  Inputs=|+-
  Sum{3..4,6,8,10,12} (6 alike) : Sum  Inputs=++|
  Sum13 : Sum  Inputs=|++
  i_tau : Outport
  wires:
  Sum8/1 -> Mux6/3
  Sum4/1 -> Mux6/5
  Sum6/1 -> Mux6/4
  Sum3/1 -> Mux6/6
  Sum12/1 -> Mux6/1
  Sum10/1 -> Mux6/2
  Derivative/1 -> Kd/1
  Kp/1 -> Sum3/2
  Kd/1 -> Sum3/1
  Sum1/1 -> Derivative/1, Kp/1
  Sum2/1 -> Kp1/1, Derivative1/1
  Kd1/1 -> Sum4/1
  Kp1/1 -> Sum4/2
  Derivative1/1 -> Kd1/1
  Derivative2/1 -> Kd2/1
  Kp2/1 -> Sum6/2
  Kd2/1 -> Sum6/1
  Sum5/1 -> Derivative2/1, Kp2/1
  Derivative3/1 -> Kd3/1
  Kp3/1 -> Sum8/2
  Kd3/1 -> Sum8/1
  Sum7/1 -> Derivative3/1, Kp3/1
  Derivative4/1 -> Kd4/1
  Kp4/1 -> Sum10/2
  Kd4/1 -> Sum10/1
  Sum9/1 -> Derivative4/1, Kp4/1
  Derivative5/1 -> Kd5/1
  Kp5/1 -> Sum12/2
  Kd5/1 -> Sum12/1
  Sum11/1 -> Derivative5/1, Kp5/1
  current/1 -> Demux1/1
  Demux1/1 -> Sum11/2
  set point/1 -> Demux/1
  Demux/1 -> Sum11/1
  Demux/2 -> Sum9/1
  Demux1/2 -> Sum9/2
  Demux/3 -> Sum7/1
  Demux1/3 -> Sum7/2
  Demux/4 -> Sum5/1
  Demux1/4 -> Sum5/2, MATLAB Function1/1(phi)
  Demux/5 -> Sum2/1
  Demux1/5 -> MATLAB Function1/2(theta), Sum2/2
  Demux/6 -> Sum1/1
  Demux1/6 -> MATLAB Function1/3(unused), Sum1/2
  MATLAB Function1/1(g_eta) -> Sum13/2  "g_eta"
  Mux6/1 -> Sum13/1  "pd_out"
  Sum13/1 -> i_tau/1

== system comparing_controllers/PD Gravity Compensated Controller/6 DOF PD Gravity Comp Controller/Subsystem ==
  ideal_t_sat : Inport
  MATLAB Function : MATLAB Function  TreatAsAtomicUnit=on
  Saturation3 : Saturate  Commented=on  UpperLimit=35  LowerLimit=-35
  rx_h : Constant  Value=0.1867
  rx_v : Constant  Value=0.0395
  ry_h : Constant  Value=0.2347
  ry_v : Constant  Value=0.2384
  rz_h : Constant  Value=0.0175
  rz_v : Constant  Value=0.0404
  theta : Constant  Value=pi/4
  tau : Outport
  wires:
  ry_v/1 -> MATLAB Function/4(ry_v)
  theta/1 -> MATLAB Function/2(theta)
  MATLAB Function/1(tau) -> tau/1
  rx_v/1 -> MATLAB Function/3(rx_v)
  ry_h/1 -> MATLAB Function/7(ry_h)
  rx_h/1 -> MATLAB Function/6(rx_h)
  rz_v/1 -> MATLAB Function/5(unused)
  ideal_t_sat/1 -> MATLAB Function/1(thrust)
  rz_h/1 -> MATLAB Function/8(rz_h)

== system comparing_controllers/PD Gravity Compensated Controller/6 DOF PD Gravity Comp Controller/Subsystem3 ==
  In1 : Inport
  NED : Inport  Port=2
  Demux : Demux  Outputs=2
  Demux1 : Demux  Outputs=2
  Demux{2..5} (4 alike) : Demux  Outputs=3
  Mux : Mux  Inputs=6
  Mux1 : Mux  Inputs=6
  Subsystem1 : Subsystem
  Subsystem2 : Subsystem
  Terminator4 : Terminator
  Terminator5 : Terminator
  Out1 : Outport
  Out2 : Outport  Port=2
  wires:
  Mux1/1 -> Out2/1
  Demux/1 -> Terminator4/1
  Demux/2 -> Demux4/1
  Demux4/3 -> Mux/6
  Demux3/2 -> Mux/2
  Demux4/2 -> Mux/5
  Demux3/3 -> Mux/3
  NED/1 -> Subsystem1/1(NED), Demux1/1
  Demux2/3 -> Mux1/3
  Subsystem1/1(pos_body) -> Demux2/1
  Demux3/1 -> Mux/1
  Mux/1 -> Out1/1
  Subsystem2/1(pos_body) -> Demux3/1
  Demux5/2 -> Mux1/5
  Demux1/2 -> Demux5/1
  Demux2/2 -> Mux1/2
  Demux5/3 -> Mux1/6
  In1/1 -> Demux/1, Subsystem2/1(NED)
  Demux1/1 -> Terminator5/1
  Demux4/1 -> Mux/4
  Demux2/1 -> Mux1/1
  Demux5/1 -> Mux1/4

== system comparing_controllers/PD Gravity Compensated Controller/6 DOF PD Gravity Comp Controller/Thrust allocation ==
  ideal_tau : Inport
  Demux6 : Demux  Commented=on  Outputs=3
  MATLAB Function : MATLAB Function  Commented=on  TreatAsAtomicUnit=on
  MATLAB Function1 : MATLAB Function  TreatAsAtomicUnit=on
  Mux2 : Mux  Commented=on  Inputs=3
  Saturation : Saturate  Commented=on  UpperLimit=70  LowerLimit=-70
  Saturation1 : Saturate  Commented=on  UpperLimit=100  LowerLimit=-100
  Saturation2 : Saturate  Commented=on  UpperLimit=100  LowerLimit=-100
  Saturation3 : Saturate  UpperLimit=35  LowerLimit=-35
  alpha : Constant  Value=pi/4
  rx_h : Constant  Value=0.1867
  rx_v : Constant  Value=0.0395
  ry_h : Constant  Value=0.2347
  ry_v : Constant  Value=0.2384
  rz_h : Constant  Value=0.0175
  rz_v : Constant  Value=0.0404
  tau : Outport
  wires:
  ideal_tau/1 -> MATLAB Function1/1(tau)  "ideal_t_sat"
  MATLAB Function1/1(thrust) -> Saturation3/1
  Saturation3/1 -> tau/1
  rx_v/1 -> MATLAB Function1/3(rx_v)
  alpha/1 -> MATLAB Function1/2(alpha)
  rx_h/1 -> MATLAB Function1/6(rx_h)
  ry_h/1 -> MATLAB Function1/7(ry_h)
  rz_h/1 -> MATLAB Function1/8(rz_h)
  ry_v/1 -> MATLAB Function1/4(ry_v)
  rz_v/1 -> MATLAB Function1/5(unused)
  Demux6/2 -> Saturation2/1
  Demux6/3 -> Saturation/1
  Saturation1/1 -> Mux2/1
  Saturation/1 -> Mux2/3
  Demux6/1 -> Saturation1/1
  Saturation2/1 -> Mux2/2

== system comparing_controllers/PD Gravity Compensated Controller/6 DOF PD Gravity Comp Controller/Transform ==
  In1 : Inport
  NED : Inport  Port=2
  Demux : Demux  Outputs=2
  Demux1 : Demux  Outputs=2
  Mux1 : Mux  Inputs=2
  Mux2 : Mux  Inputs=2
  Mux3 : Mux  Inputs=2
  Subsystem1 : Subsystem
  Subsystem2 : Subsystem
  Terminator5 : Terminator
  Out1 : Outport
  Out2 : Outport  Port=2
  wires:
  Demux/1 -> Mux2/1
  NED/1 -> Demux1/1, Subsystem1/1(NED)
  In1/1 -> Demux/1
  Demux/2 -> Mux1/2
  Subsystem2/1(pos_body) -> Mux1/1
  Demux1/1 -> Terminator5/1
  Subsystem1/1(pos_body) -> Mux3/1
  Demux1/2 -> Mux2/2, Mux3/2
  Mux2/1 -> Subsystem2/1(NED)
  Mux3/1 -> Out2/1
  Mux1/1 -> Out1/1

== system comparing_controllers/PD Gravity Compensated Controller/UUV 6DOF Model/Subsystem ==
  f : Inport
  MATLAB Function1 : MATLAB Function  TreatAsAtomicUnit=on
  rx_h : Constant  Value=0.1867
  rx_v : Constant  Value=0.0395
  ry_h : Constant  Value=0.2347
  ry_v : Constant  Value=0.2384
  rz_h : Constant  Value=0.0175
  rz_v : Constant  Value=0.0404
  theta : Constant  Value=pi/4
  tau : Outport
  wires:
  rz_v/1 -> MATLAB Function1/5(unused)
  ry_h/1 -> MATLAB Function1/7(ry_h)
  f/1 -> MATLAB Function1/1(f)
  MATLAB Function1/1(tau) -> tau/1
  rx_h/1 -> MATLAB Function1/6(rx_h)
  theta/1 -> MATLAB Function1/2(theta)
  rx_v/1 -> MATLAB Function1/3(rx_v)
  rz_h/1 -> MATLAB Function1/8(rz_h)
  ry_v/1 -> MATLAB Function1/4(ry_v)

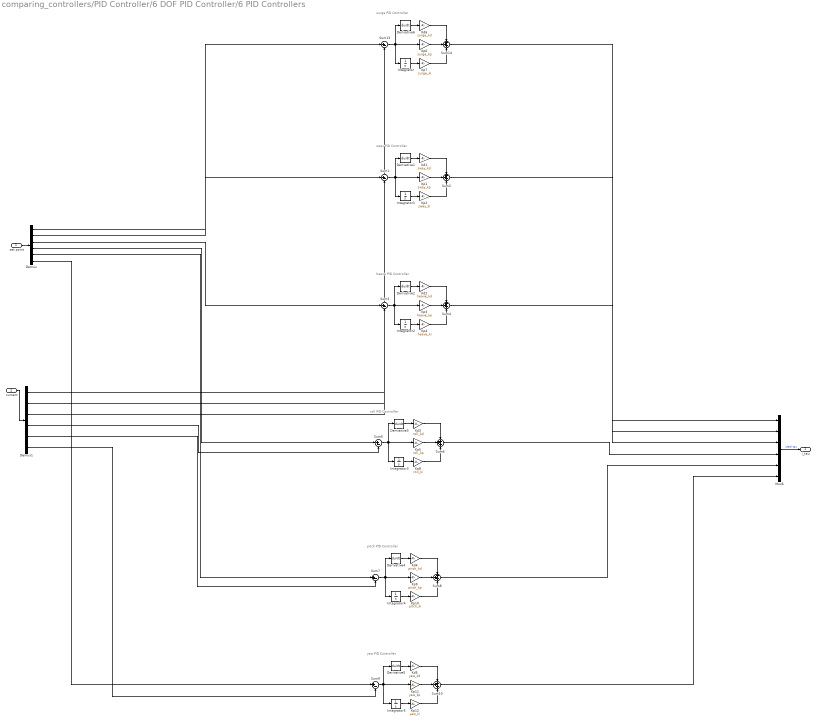
== system comparing_controllers/PID Controller/6 DOF PID Controller/6 PID Controllers ==
  note: yaw PID Controller
  note: pitch PID Controller
  note: roll PID Controller
  note: heave PID Controller
  note: sway PID Controller
  note: surge PID Controller
  set point : Inport
  current : Inport  Port=2
  Demux : Demux  Outputs=6
  Demux1 : Demux  Outputs=6
  Derivative{1..6} (6 alike) : Derivative
  Integrator{,1..5} (6 alike) : Integrator
  Kd1 : Gain  Gain=sway_kd
  Kd2 : Gain  Gain=heave_kd
  Kd3 : Gain  Gain=roll_kd
  Kd4 : Gain  Gain=pitch_kd
  Kd5 : Gain  Gain=yaw_kd
  Kd6 : Gain  Gain=surge_kd
  Kp1 : Gain  Gain=sway_kp
  Kp10 : Gain  Gain=pitch_ki
  Kp11 : Gain  Gain=yaw_kp
  Kp12 : Gain  Gain=yaw_ki
  Kp2 : Gain  Gain=sway_ki
  Kp3 : Gain  Gain=heave_kp
  Kp4 : Gain  Gain=heave_ki
  Kp5 : Gain  Gain=roll_kp
  Kp6 : Gain  Gain=surge_kp
  Kp7 : Gain  Gain=surge_ki
  Kp8 : Gain  Gain=roll_ki
  Kp9 : Gain  Gain=pitch_kp
  Mux6 : Mux  Inputs=6
  Sum{1,3,5,7,9,13} (6 alike) : Sum  Inputs=|+-
  Sum{2,4,6,8,10,14} (6 alike) : Sum  Inputs=+++
  i_tau : Outport
  wires:
  Sum4/1 -> Mux6/3
  Sum8/1 -> Mux6/5
  Sum6/1 -> Mux6/4
  Sum10/1 -> Mux6/6
  Sum14/1 -> Mux6/1
  Sum2/1 -> Mux6/2
  current/1 -> Demux1/1
  set point/1 -> Demux/1
  Mux6/1 -> i_tau/1  "ideal tau"
  Demux1/1 -> Sum13/2
  Demux/1 -> Sum13/1
  Kp7/1 -> Sum14/3
  Integrator/1 -> Kp7/1
  Kp6/1 -> Sum14/2
  Kd6/1 -> Sum14/1
  Derivative6/1 -> Kd6/1
  Sum13/1 -> Integrator/1, Derivative6/1, Kp6/1
  Demux1/2 -> Sum1/2
  Demux/2 -> Sum1/1
  Kp2/1 -> Sum2/3
  Integrator1/1 -> Kp2/1
  Kp1/1 -> Sum2/2
  Kd1/1 -> Sum2/1
  Derivative1/1 -> Kd1/1
  Sum1/1 -> Integrator1/1, Derivative1/1, Kp1/1
  Demux1/3 -> Sum3/2
  Demux/3 -> Sum3/1
  Kp4/1 -> Sum4/3
  Integrator2/1 -> Kp4/1
  Kp3/1 -> Sum4/2
  Kd2/1 -> Sum4/1
  Derivative2/1 -> Kd2/1
  Sum3/1 -> Integrator2/1, Derivative2/1, Kp3/1
  Demux1/4 -> Sum5/2
  Demux/4 -> Sum5/1
  Kp8/1 -> Sum6/3
  Integrator3/1 -> Kp8/1
  Kp5/1 -> Sum6/2
  Kd3/1 -> Sum6/1
  Derivative3/1 -> Kd3/1
  Sum5/1 -> Integrator3/1, Derivative3/1, Kp5/1
  Demux1/5 -> Sum7/2
  Demux/5 -> Sum7/1
  Kp10/1 -> Sum8/3
  Integrator4/1 -> Kp10/1
  Kp9/1 -> Sum8/2
  Kd4/1 -> Sum8/1
  Derivative4/1 -> Kd4/1
  Sum7/1 -> Integrator4/1, Derivative4/1, Kp9/1
  Demux1/6 -> Sum9/2
  Demux/6 -> Sum9/1
  Kp12/1 -> Sum10/3
  Integrator5/1 -> Kp12/1
  Kp11/1 -> Sum10/2
  Kd5/1 -> Sum10/1
  Derivative5/1 -> Kd5/1
  Sum9/1 -> Integrator5/1, Derivative5/1, Kp11/1

== system comparing_controllers/PID Controller/6 DOF PID Controller/Thrust allocation ==
  ideal_tau : Inport
  Demux6 : Demux  Commented=on  Outputs=3
  MATLAB Function : MATLAB Function  Commented=on  TreatAsAtomicUnit=on
  MATLAB Function1 : MATLAB Function  TreatAsAtomicUnit=on
  Mux2 : Mux  Commented=on  Inputs=3
  Saturation : Saturate  Commented=on  UpperLimit=70  LowerLimit=-70
  Saturation1 : Saturate  Commented=on  UpperLimit=100  LowerLimit=-100
  Saturation2 : Saturate  Commented=on  UpperLimit=100  LowerLimit=-100
  Saturation3 : Saturate  UpperLimit=35  LowerLimit=-35
  alpha : Constant  Value=pi/4
  rx_h : Constant  Value=0.1867
  rx_v : Constant  Value=0.0395
  ry_h : Constant  Value=0.2347
  ry_v : Constant  Value=0.2384
  rz_h : Constant  Value=0.0175
  rz_v : Constant  Value=0.0404
  tau : Outport
  wires:
  ideal_tau/1 -> MATLAB Function1/1(tau)  "ideal_t_sat"
  MATLAB Function1/1(thrust) -> Saturation3/1
  Saturation3/1 -> tau/1
  rx_v/1 -> MATLAB Function1/3(rx_v)
  alpha/1 -> MATLAB Function1/2(alpha)
  rx_h/1 -> MATLAB Function1/6(rx_h)
  ry_h/1 -> MATLAB Function1/7(ry_h)
  rz_h/1 -> MATLAB Function1/8(rz_h)
  ry_v/1 -> MATLAB Function1/4(ry_v)
  rz_v/1 -> MATLAB Function1/5(unused)
  Demux6/2 -> Saturation2/1
  Demux6/3 -> Saturation/1
  Saturation1/1 -> Mux2/1
  Saturation/1 -> Mux2/3
  Demux6/1 -> Saturation1/1
  Saturation2/1 -> Mux2/2

== system comparing_controllers/PID Controller/6 DOF PID Controller/Transform ==
  set point : Inport
  NED : Inport  Port=2
  Demux : Demux  Outputs=2
  Demux1 : Demux  Outputs=2
  Mux1 : Mux  Inputs=2
  Mux2 : Mux  Inputs=2
  Mux3 : Mux  Inputs=2
  Subsystem1 : Subsystem
  Subsystem2 : Subsystem
  Terminator5 : Terminator
  Out1 : Outport
  Out2 : Outport  Port=2
  wires:
  Demux/1 -> Mux2/1
  NED/1 -> Demux1/1, Subsystem1/1(NED)
  set point/1 -> Demux/1
  Demux/2 -> Mux1/2
  Subsystem2/1(pos_body) -> Mux1/1
  Demux1/1 -> Terminator5/1
  Subsystem1/1(pos_body) -> Mux3/1
  Demux1/2 -> Mux2/2, Mux3/2
  Mux2/1 -> Subsystem2/1(NED)
  Mux3/1 -> Out2/1
  Mux1/1 -> Out1/1

== system comparing_controllers/PID Controller/UUV 6DOF Model/Subsystem ==
  f : Inport
  MATLAB Function1 : MATLAB Function  TreatAsAtomicUnit=on
  rx_h : Constant  Value=0.1867
  rx_v : Constant  Value=0.0395
  ry_h : Constant  Value=0.2347
  ry_v : Constant  Value=0.2384
  rz_h : Constant  Value=0.0175
  rz_v : Constant  Value=0.0404
  theta : Constant  Value=pi/4
  tau : Outport
  wires:
  rz_v/1 -> MATLAB Function1/5(unused)
  ry_h/1 -> MATLAB Function1/7(ry_h)
  f/1 -> MATLAB Function1/1(f)
  MATLAB Function1/1(tau) -> tau/1
  rx_h/1 -> MATLAB Function1/6(rx_h)
  theta/1 -> MATLAB Function1/2(theta)
  rx_v/1 -> MATLAB Function1/3(rx_v)
  rz_h/1 -> MATLAB Function1/8(rz_h)
  ry_v/1 -> MATLAB Function1/4(ry_v)

== system comparing_controllers/Computed Torque/Computed Torque Controller/Transform/Subsystem1 ==
  NED : Inport
  Demux : Demux  Outputs=2
  Demux1 : Demux  Outputs=3
  Derivative : Derivative  Commented=on
  Invert 3x3 Matrix : aerolibutil/Invert  3x3 Matrix
  Invert 3x3 Matrix1 : aerolibutil/Invert  3x3 Matrix  Commented=on
  MatrixMultiply : Product  Commented=on  Multiplication=Matrix(*)
  MatrixMultiply1 : Product  Multiplication=Matrix(*)
  Mux1 : Mux  Inputs=3
  Rzxy : Subsystem
  T : Subsystem  Commented=on
  Terminator : Terminator  Commented=on
  pos_body : Outport
  wires:
  Demux1/2 -> Mux1/2, T/2(In2)  "theta"
  Demux1/1 -> Mux1/1, T/1(In1)  "phi"
  Rzxy/1(J) -> Invert 3x3 Matrix/1
  Mux1/1 -> Derivative/1, Rzxy/1(angles)
  Derivative/1 -> MatrixMultiply/2  "euler_dot"
  Invert 3x3 Matrix1/1 -> MatrixMultiply/1  "T'"
  Demux1/3 -> Mux1/3  "psi"
  MatrixMultiply/1 -> Terminator/1  "ang_vel_body"
  T/1(T) -> Invert 3x3 Matrix1/1
  Invert 3x3 Matrix/1 -> MatrixMultiply1/1  "R'"
  MatrixMultiply1/1 -> pos_body/1
  NED/1 -> Demux/1
  Demux/2 -> Demux1/1
  Demux/1 -> MatrixMultiply1/2

== system comparing_controllers/Computed Torque/Computed Torque Controller/Transform/Subsystem2 ==
  NED : Inport
  Demux : Demux  Outputs=2
  Demux1 : Demux  Outputs=3
  Derivative : Derivative  Commented=on
  Invert 3x3 Matrix : aerolibutil/Invert  3x3 Matrix
  Invert 3x3 Matrix1 : aerolibutil/Invert  3x3 Matrix  Commented=on
  MatrixMultiply : Product  Commented=on  Multiplication=Matrix(*)
  MatrixMultiply1 : Product  Multiplication=Matrix(*)
  Mux1 : Mux  Inputs=3
  Rzxy : Subsystem
  T : Subsystem  Commented=on
  Terminator : Terminator  Commented=on
  pos_body : Outport
  wires:
  Demux1/2 -> Mux1/2, T/2(In2)  "theta"
  Demux1/1 -> Mux1/1, T/1(In1)  "phi"
  Rzxy/1(J) -> Invert 3x3 Matrix/1
  Mux1/1 -> Derivative/1, Rzxy/1(angles)
  Derivative/1 -> MatrixMultiply/2  "euler_dot"
  Invert 3x3 Matrix1/1 -> MatrixMultiply/1  "T'"
  Demux1/3 -> Mux1/3  "psi"
  MatrixMultiply/1 -> Terminator/1  "ang_vel_body"
  T/1(T) -> Invert 3x3 Matrix1/1
  Invert 3x3 Matrix/1 -> MatrixMultiply1/1  "R'"
  MatrixMultiply1/1 -> pos_body/1
  NED/1 -> Demux/1
  Demux/2 -> Demux1/1
  Demux/1 -> MatrixMultiply1/2

== system comparing_controllers/PD Controller/6 DOF PD Controller/Transform/Subsystem1 ==
  NED : Inport
  Demux : Demux  Outputs=2
  Demux1 : Demux  Outputs=3
  Derivative : Derivative  Commented=on
  Invert 3x3 Matrix : aerolibutil/Invert  3x3 Matrix
  Invert 3x3 Matrix1 : aerolibutil/Invert  3x3 Matrix  Commented=on
  MatrixMultiply : Product  Commented=on  Multiplication=Matrix(*)
  MatrixMultiply1 : Product  Multiplication=Matrix(*)
  Mux1 : Mux  Inputs=3
  Rzxy : Subsystem
  T : Subsystem  Commented=on
  Terminator : Terminator  Commented=on
  pos_body : Outport
  wires:
  Demux1/2 -> Mux1/2, T/2(In2)  "theta"
  Demux1/1 -> Mux1/1, T/1(In1)  "phi"
  Rzxy/1(J) -> Invert 3x3 Matrix/1
  Mux1/1 -> Derivative/1, Rzxy/1(angles)
  Derivative/1 -> MatrixMultiply/2  "euler_dot"
  Invert 3x3 Matrix1/1 -> MatrixMultiply/1  "T'"
  Demux1/3 -> Mux1/3  "psi"
  MatrixMultiply/1 -> Terminator/1  "ang_vel_body"
  T/1(T) -> Invert 3x3 Matrix1/1
  Invert 3x3 Matrix/1 -> MatrixMultiply1/1  "R'"
  MatrixMultiply1/1 -> pos_body/1
  NED/1 -> Demux/1
  Demux/2 -> Demux1/1
  Demux/1 -> MatrixMultiply1/2

== system comparing_controllers/PD Controller/6 DOF PD Controller/Transform/Subsystem2 ==
  NED : Inport
  Demux : Demux  Outputs=2
  Demux1 : Demux  Outputs=3
  Derivative : Derivative  Commented=on
  Invert 3x3 Matrix : aerolibutil/Invert  3x3 Matrix
  Invert 3x3 Matrix1 : aerolibutil/Invert  3x3 Matrix  Commented=on
  MatrixMultiply : Product  Commented=on  Multiplication=Matrix(*)
  MatrixMultiply1 : Product  Multiplication=Matrix(*)
  Mux1 : Mux  Inputs=3
  Rzxy : Subsystem
  T : Subsystem  Commented=on
  Terminator : Terminator  Commented=on
  pos_body : Outport
  wires:
  Demux1/2 -> Mux1/2, T/2(In2)  "theta"
  Demux1/1 -> Mux1/1, T/1(In1)  "phi"
  Rzxy/1(J) -> Invert 3x3 Matrix/1
  Mux1/1 -> Derivative/1, Rzxy/1(angles)
  Derivative/1 -> MatrixMultiply/2  "euler_dot"
  Invert 3x3 Matrix1/1 -> MatrixMultiply/1  "T'"
  Demux1/3 -> Mux1/3  "psi"
  MatrixMultiply/1 -> Terminator/1  "ang_vel_body"
  T/1(T) -> Invert 3x3 Matrix1/1
  Invert 3x3 Matrix/1 -> MatrixMultiply1/1  "R'"
  MatrixMultiply1/1 -> pos_body/1
  NED/1 -> Demux/1
  Demux/2 -> Demux1/1
  Demux/1 -> MatrixMultiply1/2
